simulink library "MOST_Lib"  (R2020b)
settings: Solver=VariableStepAuto  StartTime=0.0  StopTime=10.0  RelTol=1e-3
undefined symbols (not defined in the file): simu, wind, windTurbine, windturbine, X, Y, Z
libraries: nesl_utility x54, sm_lib x50, simulink x4, simulink_extras x1, pid_lib x1, WECSim_Lib_Body_Elements x1
(part 2 of 3)

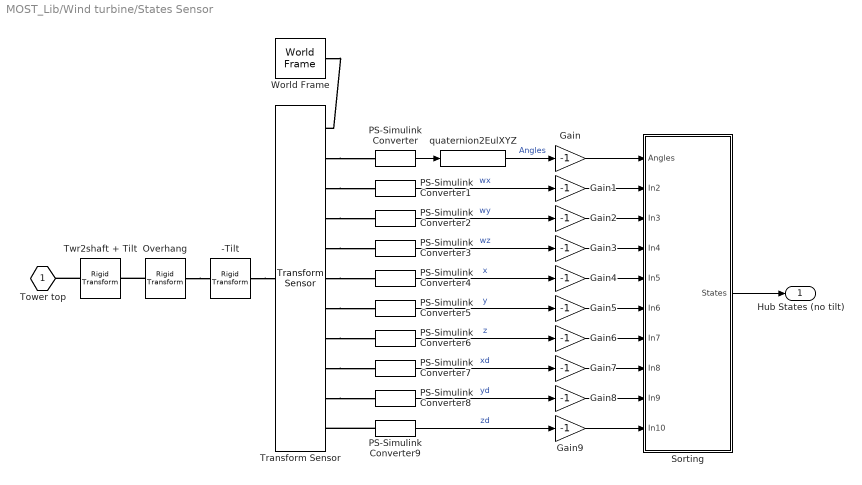
== system MOST_Lib/Wind turbine/States Sensor ==
  -Tilt : sm_lib/Frames and Transforms/Rigid Transform  RotationMethod=StandardAxis  FollAlignAxisA=+X  BaseAlignAxisA=+Y  FollAlignAxisB=+Y  BaseAlignAxisB=+Z  RotationStandardAxis=+Y  RotationAngle=-windTurbine.nacelle.tiltangle  RotationAngleUnits=deg  RotationArbitraryAxis=[0 0 1]  RotationSequenceAxes=FollowerAxes  RotationSequence=XYX  RotationSequenceAngles=[0 0 0]  RotationSequenceAnglesUnits=deg  RotationMatrix=[1 0 0; 0 1 0; 0 0 1]  Quaternion=[1 0 0 0]  TranslationMethod=None  TranslationCartesianOffset=[0 0 0]  TranslationCartesianOffsetUnits=m  TranslationStandardAxis=+Z  TranslationStandardOffset=0  TranslationStandardOffsetUnits=m  TranslationROffset=0  TranslationROffsetUnits=m  TranslationThetaOffset=0  TranslationThetaOffsetUnits=deg  TranslationZOffset=0  TranslationZOffsetUnits=m
  Gain{,1..9} (10 alike) : Gain  Gain=-1
  Overhang : sm_lib/Frames and Transforms/Rigid Transform  RotationMethod=None  FollAlignAxisA=+X  BaseAlignAxisA=+Y  FollAlignAxisB=+Y  BaseAlignAxisB=+Z  RotationStandardAxis=+Z  RotationAngle=0.0  RotationAngleUnits=deg  RotationArbitraryAxis=[0 0 1]  RotationSequenceAxes=FollowerAxes  RotationSequence=XYX  RotationSequenceAngles=[0 0 0]  RotationSequenceAnglesUnits=deg  RotationMatrix=[1 0 0; 0 1 0; 0 0 1]  Quaternion=[1 0 0 0]  TranslationMethod=StandardAxis  TranslationCartesianOffset=[0 0 0]  TranslationCartesianOffsetUnits=m  TranslationStandardAxis=+X  TranslationStandardOffset=windTurbine.hub.overhang  TranslationStandardOffsetUnits=m  TranslationROffset=0  TranslationROffsetUnits=m  TranslationThetaOffset=0  TranslationThetaOffsetUnits=deg  TranslationZOffset=0  TranslationZOffsetUnits=m
  PS-Simulink Converter{,1..9} (10 alike) : nesl_utility/PS-Simulink Converter  PhysicalDomain=network_engine_domain  SubClassName=ps_output  LeftPortType=input  RightPortType=output  PseudoPeriodic=off  Frequencies=[]  VectorFormat=inherit  Unit=inherit  AffineConversion=off
  Sorting : Subsystem
  Transform Sensor : sm_lib/Frames and Transforms/Transform Sensor  MeasurementFrame=World  RotationSequence=XYZ  SenseAngle=off  SenseAxis=off  SenseQ=on  SenseR=off  SenseRotationSequence=off  SenseOmegaX=on  SenseOmegaY=on  SenseOmegaZ=on  SenseOmega=off  SenseQDot=off  SenseRDot=off  SenseRotationSequenceDot=off  SenseAlphaX=off  SenseAlphaY=off  SenseAlphaZ=off  SenseAlpha=off  SenseQDDot=off  SenseRDDot=off  SenseX=on  SenseY=on  SenseZ=on  SenseXYZ=off  SenseRad=off  SenseAzim=off  SenseDist=off  SenseInc=off  SenseXDot=on  SenseYDot=on  SenseZDot=on  SenseXYZDot=off  SenseRadDot=off  SenseAzimDot=off  SenseDistDot=off  SenseIncDot=off  SenseXDDot=off  SenseYDDot=off  SenseZDDot=off  SenseXYZDDot=off  SenseRadDDot=off  SenseAzimDDot=off  SenseDistDDot=off  SenseIncDDot=off
  "Twr2shaft + Tilt " : sm_lib/Frames and Transforms/Rigid Transform  RotationMethod=StandardAxis  FollAlignAxisA=+X  BaseAlignAxisA=+Y  FollAlignAxisB=+Y  BaseAlignAxisB=+Z  RotationStandardAxis=+Y  RotationAngle=windTurbine.nacelle.tiltangle  RotationAngleUnits=deg  RotationArbitraryAxis=[0 0 1]  RotationSequenceAxes=FollowerAxes  RotationSequence=XYX  RotationSequenceAngles=[0 0 0]  RotationSequenceAnglesUnits=deg  RotationMatrix=[1 0 0; 0 1 0; 0 0 1]  Quaternion=[1 0 0 0]  TranslationMethod=StandardAxis  TranslationCartesianOffset=[0 0 0]  TranslationCartesianOffsetUnits=m  TranslationStandardAxis=+Z  TranslationStandardOffset=windTurbine.nacelle.Twr2Shft  TranslationStandardOffsetUnits=m  TranslationROffset=0  TranslationROffsetUnits=m  TranslationThetaOffset=0  TranslationThetaOffsetUnits=deg  TranslationZOffset=0  TranslationZOffsetUnits=m
  World Frame : sm_lib/Frames and Transforms/World Frame
  quaternion2EulXYZ : WECSim_Lib_Body_Elements/Rigid Body/Hydrodynamic Body/Structure/Motion Sensor/quaternion2EulXYZ  SystemSampleTime=-1  VariantActivationTime=update diagram  Latency=0  AutoFrameSizeCalculation=off
  Tower top : PMIOPort  Side=Left
  Hub States (no tilt) : Outport
  wires:
  PS-Simulink Converter/1 -> quaternion2EulXYZ/1
  quaternion2EulXYZ/1 -> Gain/1  "Angles"
  PS-Simulink Converter1/1 -> Gain1/1  "wx"
  PS-Simulink Converter2/1 -> Gain2/1  "wy"
  PS-Simulink Converter3/1 -> Gain3/1  "wz"
  PS-Simulink Converter4/1 -> Gain4/1  "x"
  PS-Simulink Converter5/1 -> Gain5/1  "y"
  PS-Simulink Converter6/1 -> Gain6/1  "z"
  PS-Simulink Converter7/1 -> Gain7/1  "xd"
  PS-Simulink Converter8/1 -> Gain8/1  "yd"
  PS-Simulink Converter9/1 -> Gain9/1  "zd"
  Sorting/1(States) -> Hub States (no tilt)/1
  Gain/1 -> Sorting/1(Angles)
  Gain1/1 -> Sorting/2(In2)
  Gain2/1 -> Sorting/3(In3)
  Gain3/1 -> Sorting/4(In4)
  Gain4/1 -> Sorting/5(In5)
  Gain5/1 -> Sorting/6(In6)
  Gain6/1 -> Sorting/7(In7)
  Gain7/1 -> Sorting/8(In8)
  Gain8/1 -> Sorting/9(In9)
  Gain9/1 -> Sorting/10(In10)
  connections:
  Transform Sensor/RConn7 -- PS-Simulink Converter5/LConn1
  World Frame/RConn1 -- Transform Sensor/RConn1
  "Twr2shaft + Tilt "/LConn1 -- Tower top/RConn1
  Transform Sensor/RConn2 -- PS-Simulink Converter/LConn1
  Transform Sensor/RConn3 -- PS-Simulink Converter1/LConn1
  Transform Sensor/RConn4 -- PS-Simulink Converter2/LConn1
  Transform Sensor/RConn5 -- PS-Simulink Converter3/LConn1
  Transform Sensor/RConn6 -- PS-Simulink Converter4/LConn1
  Transform Sensor/RConn9 -- PS-Simulink Converter7/LConn1
  Transform Sensor/RConn8 -- PS-Simulink Converter6/LConn1
  Transform Sensor/RConn10 -- PS-Simulink Converter8/LConn1
  PS-Simulink Converter9/LConn1 -- Transform Sensor/RConn11
  -Tilt/RConn1 -- Transform Sensor/LConn1
  Overhang/RConn1 -- -Tilt/LConn1
  Overhang/LConn1 -- "Twr2shaft + Tilt "/RConn1

== system MOST_Lib/Wind turbine/Tower ==
  Body Properties Tower : sm_lib/Body Elements/File Solid  ExtGeomFileName=geometry/NREL5MW_Tower.STL  UnitType=Custom  ExtGeomFileUnits=m  StepReaderType=HEX  ExportConvexHullGeometry=off  InertiaType=Custom  BasedOnType=Density  Density=1000  DensityUnits=kg/(m^3)  Mass=windTurbine.tower.mass  MassUnits=kg  CenterOfMass=[0 0 0]  CenterOfMassUnits=m  MomentsOfInertia=windTurbine.tower.inertia  MomentsOfInertiaUnits=kg*m^2  ProductsOfInertia=windTurbine.tower.inertiaProducts  ProductsOfInertiaUnits=kg*m^2  GraphicType=FromGeometry  MarkerShape=Sphere  MarkerSize=10  GraphicVisPropType=SimpleVisualProperties  GraphicDiffuseColor=[1 1 1]  GraphicOpacity=1  GraphicSpecularColor=[0.5 0.5 0.5 1.0]  GraphicAmbientColor=[0.15 0.15 0.15 1.0]  GraphicEmissiveColor=[0.0 0.0 0.0 1.0]  GraphicShininess=75  DoExposeReferenceFrame=on  SerializedFrames=<Frames/>
  Constant : Constant  Value=-windTurbine.tower.mass*simu.gravity
  External Force and Torque : sm_lib/Forces and Torques/External Force and Torque  EnableForceX=off  EnableForceY=off  EnableForceZ=on  EnableForce=off  ForceResolutionFrame=World  EnableTorqueX=off  EnableTorqueY=off  EnableTorqueZ=off  EnableTorque=off  TorqueResolutionFrame=AttachedFrame
  Relative COG Tower : sm_lib/Frames and Transforms/Rigid Transform  RotationMethod=None  FollAlignAxisA=+X  BaseAlignAxisA=+Y  FollAlignAxisB=+Y  BaseAlignAxisB=+Z  RotationStandardAxis=+Y  RotationAngle=0.05  RotationAngleUnits=rad  RotationArbitraryAxis=[0.57735026918962584 0.57735026918962584 0.57735026918962584]  RotationSequenceAxes=FollowerAxes  RotationSequence=XYX  RotationSequenceAngles=[0 0 0]  RotationSequenceAnglesUnits=deg  RotationMatrix=[1 0 0; 0 1 0; 0 0 1]  Quaternion=[1 0 0 0]  TranslationMethod=Cartesian  TranslationCartesianOffset=windTurbine.tower.cog_rel  TranslationCartesianOffsetUnits=m  TranslationStandardAxis=+Z  TranslationStandardOffset=0  TranslationStandardOffsetUnits=m  TranslationROffset=0  TranslationROffsetUnits=m  TranslationThetaOffset=0  TranslationThetaOffsetUnits=deg  TranslationZOffset=0  TranslationZOffsetUnits=m
  Simulink-PS Converter : nesl_utility/Simulink-PS Converter  PhysicalDomain=network_engine_domain  SubClassName=ps_input  LeftPortType=input  RightPortType=output  PseudoPeriodic=off  Frequencies=[]  NoiseDistribution=none  NoiseParameters=[]  Unit=1  AffineConversion=off  FilteringAndDerivatives=provide  SimscapeFilterOrder=1  InputFilterTimeConstant=0.001  UdotUserProvided=0
  Tower Base : PMIOPort  Side=Left
  wires:
  Constant/1 -> Simulink-PS Converter/1
  connections:
  Simulink-PS Converter/RConn1 -- External Force and Torque/LConn1
  Relative COG Tower/LConn1 -- Tower Base/RConn1
  Body Properties Tower/RConn1 -- Relative COG Tower/RConn1 -- External Force and Torque/RConn1

== system MOST_Lib/Wind turbine/TowerBaseLoad ==
  Mux : Mux  Inputs=2
  PS-Simulink Converter6 : nesl_utility/PS-Simulink Converter  PhysicalDomain=network_engine_domain  SubClassName=ps_output  LeftPortType=input  RightPortType=output  PseudoPeriodic=off  Frequencies=[]  VectorFormat=1-D array  Unit=inherit  AffineConversion=off
  PS-Simulink Converter7 : nesl_utility/PS-Simulink Converter  PhysicalDomain=network_engine_domain  SubClassName=ps_output  LeftPortType=input  RightPortType=output  PseudoPeriodic=off  Frequencies=[]  VectorFormat=1-D array  Unit=inherit  AffineConversion=off
  fc : PMIOPort  Side=Left
  tc : PMIOPort  Port=2  Side=Left
  tag scope: TowerBaseLoad1=global
  wires:
  PS-Simulink Converter7/1 -> Mux/1
  PS-Simulink Converter6/1 -> Mux/2
  Mux/1 -> [TowerBaseLoad1]
  connections:
  fc/RConn1 -- PS-Simulink Converter7/LConn1
  tc/RConn1 -- PS-Simulink Converter6/LConn1

== system MOST_Lib/Wind turbine/TowerTopLoad and deltaYaw ==
  Mux1 : Mux  Inputs=2
  PS-Simulink Converter1 : nesl_utility/PS-Simulink Converter  PhysicalDomain=network_engine_domain  SubClassName=ps_output  LeftPortType=input  RightPortType=output  PseudoPeriodic=off  Frequencies=[]  VectorFormat=1-D array  Unit=rad  AffineConversion=off
  PS-Simulink Converter8 : nesl_utility/PS-Simulink Converter  PhysicalDomain=network_engine_domain  SubClassName=ps_output  LeftPortType=input  RightPortType=output  PseudoPeriodic=off  Frequencies=[]  VectorFormat=1-D array  Unit=inherit  AffineConversion=off
  PS-Simulink Converter9 : nesl_utility/PS-Simulink Converter  PhysicalDomain=network_engine_domain  SubClassName=ps_output  LeftPortType=input  RightPortType=output  PseudoPeriodic=off  Frequencies=[]  VectorFormat=1-D array  Unit=inherit  AffineConversion=off
  q : PMIOPort  Side=Left
  ft : PMIOPort  Port=2  Side=Left
  tt : PMIOPort  Port=3  Side=Left
  tag scope: DeltaYaw1=global, TowerTopLoad1=global
  wires:
  PS-Simulink Converter9/1 -> Mux1/1
  PS-Simulink Converter8/1 -> Mux1/2
  Mux1/1 -> [TowerTopLoad1]
  PS-Simulink Converter1/1 -> [DeltaYaw1]
  connections:
  ft/RConn1 -- PS-Simulink Converter9/LConn1
  tt/RConn1 -- PS-Simulink Converter8/LConn1
  q/RConn1 -- PS-Simulink Converter1/LConn1

== system MOST_Lib/Wind turbine/Aerodynamics + Control/Aeroloads ==
  note: 1) Add Subsystem or Model blocks as valid variant choices.
      | 2) You cannot connect blocks at this level. At simulation, connectivity is automatically
      | determined, based on the active variant and port name matching.
  Aeroloads_in : Inport
  BEM : Subsystem  VariantControl=sv_t1_AeroLoads1
  Look-up Tables : Subsystem  VariantControl=sv_t1_AeroLoads0
  F_aero : Outport

== system MOST_Lib/Wind turbine/Aerodynamics + Control/Control ==
  note: 1) Add Subsystem or Model blocks as valid variant choices.
      | 2) You cannot connect blocks at this level. At simulation, connectivity is automatically
      | determined, based on the active variant and port name matching.
  Rotor speed : Inport
  Baseline : Subsystem  VariantControl=sv_t1_control0
  ROSCO : Subsystem  VariantControl=sv_t1_control1
  Gen torque : Outport
  Bladepitch : Outport  Port=2

== system MOST_Lib/Wind turbine/Aerodynamics + Control/Yaw Control ==
  Hub states (no tilt) : Inport
  Atan : Trigonometry  Operator=atan2  OutputSignalType=real
  Constant : Constant  Value=windTurbine.YawControlFlag
  Constant1 : Constant  Value=0
  Demux : Demux  Outputs=3
  Integrator : Integrator
  PID Controller : pid_lib/PID Controller  Controller=PID  Form=Parallel  TimeDomain=Continuous-time  UseExternalTs=off  SampleTime=-1  IntegratorMethod=Forward Euler  FilterMethod=Forward Euler  ControllerParametersSource=internal  P=windTurbine.YawControl.Kp  I=windTurbine.YawControl.Ki  D=windTurbine.YawControl.Kd  N=100  UseFilter=on  TunerSelectOption=Transfer Function Based (PID Tuner App)  InitialConditionSource=internal  InitialConditionForIntegrator=0  InitialConditionForFilter=0  DifferentiatorICPrevScaledInput=0  ExternalReset=none  TrackingMode=off  Kt=1  LimitOutput=on  SatLimitsSource=internal  UpperSaturationLimit=windTurbine.YawControl.maxYawRate  LowerSaturationLimit=-windTurbine.YawControl.maxYawRate  LinearizeAsGain=on  AntiWindupMode=clamping  Kb=1  POutMin=[]  POutMax=[]  IOutMin=[]  IOutMax=[]  DOutMin=[]  DOutMax=[]  NOutMin=[]  NOutMax=[]  SumOutMin=[]  SumOutMax=[]  SaturationOutMin=[]  SaturationOutMax=[]  PParamMin=[]  PParamMax=[]  IParamMin=[]  IParamMax=[]  DParamMin=[]  DParamMax=[]  NParamMin=[]  NParamMax=[]  KbParamMin=[]  KbParamMax=[]  KtParamMin=[]  KtParamMax=[]  KbOutMin=[]  KbOutMax=[]  KtOutMin=[]  KtOutMax=[]  IntegratorOutMin=[]  IntegratorOutMax=[]  FilterOutMin=[]  FilterOutMax=[]  SumI1OutMin=[]  SumI1OutMax=[]  SumI2OutMin=[]  SumI2OutMax=[]  SumI3OutMin=[]  SumI3OutMax=[]  SumI4OutMin=[]  SumI4OutMax=[]  SumDOutMin=[]  SumDOutMax=[]  DifferentiatorOutMin=[]  DifferentiatorOutMax=[]  FilterDiffOutCoefMin=[]  FilterDiffOutCoefMax=[]  ReciprocalOutMin=[]  ReciprocalOutMax=[]  SumDenOutMin=[]  SumDenOutMax=[]  SumNumOutMin=[]  SumNumOutMax=[]  DivideOutMin=[]  DivideOutMax=[]  UdiffTsProdOutMin=[]  UdiffTsProdOutMax=[]  NTsProdOutMin=[]  NTsProdOutMax=[]  UintegralTsProdOutMin=[]  UintegralTsProdOutMax=[]  UngainTsProdOutMin=[]  UngainTsProdOutMax=[]  IntegratorContinuousStateAttributes=''  IntegratorStateMustResolveToSignalObject=off  IntegratorRTWStateStorageClass=Auto  FilterContinuousStateAttributes=''  FilterStateMustResolveToSignalObject=off  FilterRTWStateStorageClass=Auto  ParallelPVariant=InternalParameters  IdealPVariant=Disabled  IVariant=InternalParameters  DVariant=InternalParameters  IntegratorVariant=Continuous  SatVariant=Enabled  AWVariant=ContClampingParallel  PCopyVariant=Disabled  TRVariant=Disabled  FdbkBlocksVariant=Forward  IdealPFdbkVariant=Disabled  SatFdbkVariant=Disabled  DerivativeFilterVariant=ContFilter  NVariant=InternalParameters  NCopyVariant=Disabled  FilterICVariant=InternalICsFilter  IntegratorICVariant=InternalICs  ExternalResetVariant=Disabled  TRSumVariant=Passthrough  SumFdbkVariant=Disabled  SumVariant=Sum_PID  TsampFilterVariant=InternalTs  TsampNgainVariant=Passthrough  TsampIntegralVariant=Disabled_SignalSpec  ExternalSaturationOutDataTypeStr=Inherit: Same as second input
  Selector : Selector  InputPortWidth=12  IndexOptions=Index vector (dialog)  Indices=[6]  OutputSizes=1
  Sum : Sum  Inputs=+|-
  Switch : Switch  Criteria=u2 > Threshold
  Terminator : Terminator
  Transfer Fcn : TransferFcn  Denominator=[windTurbine.YawControl.tau_system 1]
  DeltaYaw : Outport
  wires:
  Hub states (no tilt)/1 -> Selector/1
  Selector/1 -> Sum/2  "Hub Yaw (fb)"
  [WindSpeed1] -> Demux/1  "m/s"
  Demux/3 -> Terminator/1
  Demux/2 -> Atan/1
  Demux/1 -> Atan/2
  Atan/1 -> Sum/1  "wind xy angle (set)"
  Integrator/1 -> Switch/1
  Transfer Fcn/1 -> Integrator/1
  PID Controller/1 -> Transfer Fcn/1
  Sum/1 -> PID Controller/1
  Constant/1 -> Switch/2
  Constant1/1 -> Switch/3
  Switch/1 -> DeltaYaw/1

== system MOST_Lib/Wind turbine/Blade 1/Blade ==
  Body Properties Blade : sm_lib/Body Elements/File Solid  ExtGeomFileName=geometry/NREL5MW_Blade.STL  UnitType=Custom  ExtGeomFileUnits=m  StepReaderType=HEX  ExportConvexHullGeometry=off  InertiaType=Custom  BasedOnType=Density  Density=1000  DensityUnits=kg/(m^3)  Mass=windTurbine.blade.mass  MassUnits=kg  CenterOfMass=[0 0 0]  CenterOfMassUnits=m  MomentsOfInertia=windTurbine.blade.inertia  MomentsOfInertiaUnits=kg*m^2  ProductsOfInertia=windTurbine.blade.inertiaProducts  ProductsOfInertiaUnits=kg*m^2  GraphicType=FromGeometry  MarkerShape=Sphere  MarkerSize=10  GraphicVisPropType=SimpleVisualProperties  GraphicDiffuseColor=[1 1 1]  GraphicOpacity=1  GraphicSpecularColor=[0.5 0.5 0.5 1.0]  GraphicAmbientColor=[0.15 0.15 0.15 1.0]  GraphicEmissiveColor=[0.0 0.0 0.0 1.0]  GraphicShininess=75  DoExposeReferenceFrame=on  SerializedFrames=<Frames/>
  Constant : Constant  Value=-windTurbine.blade.mass*simu.gravity
  External Force and Torque : sm_lib/Forces and Torques/External Force and Torque  EnableForceX=off  EnableForceY=off  EnableForceZ=on  EnableForce=off  ForceResolutionFrame=World  EnableTorqueX=off  EnableTorqueY=off  EnableTorqueZ=off  EnableTorque=off  TorqueResolutionFrame=AttachedFrame
  Relative COG Blade : sm_lib/Frames and Transforms/Rigid Transform  RotationMethod=None  FollAlignAxisA=+X  BaseAlignAxisA=+Y  FollAlignAxisB=+Y  BaseAlignAxisB=+Z  RotationStandardAxis=+Y  RotationAngle=0.05  RotationAngleUnits=rad  RotationArbitraryAxis=[0.57735026918962584 0.57735026918962584 0.57735026918962584]  RotationSequenceAxes=FollowerAxes  RotationSequence=XYX  RotationSequenceAngles=[0 0 0]  RotationSequenceAnglesUnits=deg  RotationMatrix=[1 0 0; 0 1 0; 0 0 1]  Quaternion=[1 0 0 0]  TranslationMethod=Cartesian  TranslationCartesianOffset=windTurbine.blade.cog_rel  TranslationCartesianOffsetUnits=m  TranslationStandardAxis=+Z  TranslationStandardOffset=0  TranslationStandardOffsetUnits=m  TranslationROffset=0  TranslationROffsetUnits=m  TranslationThetaOffset=0  TranslationThetaOffsetUnits=deg  TranslationZOffset=0  TranslationZOffsetUnits=m
  Simulink-PS Converter : nesl_utility/Simulink-PS Converter  PhysicalDomain=network_engine_domain  SubClassName=ps_input  LeftPortType=input  RightPortType=output  PseudoPeriodic=off  Frequencies=[]  NoiseDistribution=none  NoiseParameters=[]  Unit=1  AffineConversion=off  FilteringAndDerivatives=provide  SimscapeFilterOrder=1  InputFilterTimeConstant=0.001  UdotUserProvided=0
  Blade Root : PMIOPort  Side=Left
  wires:
  Constant/1 -> Simulink-PS Converter/1
  connections:
  Relative COG Blade/RConn1 -- Body Properties Blade/RConn1 -- External Force and Torque/RConn1
  Relative COG Blade/LConn1 -- Blade Root/RConn1
  Simulink-PS Converter/RConn1 -- External Force and Torque/LConn1

== system MOST_Lib/Wind turbine/Blade 1/bladeRootLoad ==
  Mux : Mux  Inputs=2
  PS-Simulink Converter5 : nesl_utility/PS-Simulink Converter  PhysicalDomain=network_engine_domain  SubClassName=ps_output  LeftPortType=input  RightPortType=output  PseudoPeriodic=off  Frequencies=[]  VectorFormat=1-D array  Unit=inherit  AffineConversion=off
  PS-Simulink Converter6 : nesl_utility/PS-Simulink Converter  PhysicalDomain=network_engine_domain  SubClassName=ps_output  LeftPortType=input  RightPortType=output  PseudoPeriodic=off  Frequencies=[]  VectorFormat=1-D array  Unit=inherit  AffineConversion=off
  fc : PMIOPort  Side=Left
  tc : PMIOPort  Port=2  Side=Left
  tag scope: blade1RootLoad1=global
  wires:
  PS-Simulink Converter6/1 -> Mux/2
  Mux/1 -> [blade1RootLoad1]
  PS-Simulink Converter5/1 -> Mux/1
  connections:
  tc/RConn1 -- PS-Simulink Converter6/LConn1
  fc/RConn1 -- PS-Simulink Converter5/LConn1

== system MOST_Lib/Wind turbine/Blade 2/Blade ==
  Body Properties Blade : sm_lib/Body Elements/File Solid  ExtGeomFileName=geometry/NREL5MW_Blade.STL  UnitType=Custom  ExtGeomFileUnits=m  StepReaderType=HEX  ExportConvexHullGeometry=off  InertiaType=Custom  BasedOnType=Density  Density=1000  DensityUnits=kg/(m^3)  Mass=windTurbine.blade.mass  MassUnits=kg  CenterOfMass=[0 0 0]  CenterOfMassUnits=m  MomentsOfInertia=windTurbine.blade.inertia  MomentsOfInertiaUnits=kg*m^2  ProductsOfInertia=windTurbine.blade.inertiaProducts  ProductsOfInertiaUnits=kg*m^2  GraphicType=FromGeometry  MarkerShape=Sphere  MarkerSize=10  GraphicVisPropType=SimpleVisualProperties  GraphicDiffuseColor=[1 1 1]  GraphicOpacity=1  GraphicSpecularColor=[0.5 0.5 0.5 1.0]  GraphicAmbientColor=[0.15 0.15 0.15 1.0]  GraphicEmissiveColor=[0.0 0.0 0.0 1.0]  GraphicShininess=75  DoExposeReferenceFrame=on  SerializedFrames=<Frames/>
  Constant : Constant  Value=-windTurbine.blade.mass*simu.gravity
  External Force and Torque : sm_lib/Forces and Torques/External Force and Torque  EnableForceX=off  EnableForceY=off  EnableForceZ=on  EnableForce=off  ForceResolutionFrame=World  EnableTorqueX=off  EnableTorqueY=off  EnableTorqueZ=off  EnableTorque=off  TorqueResolutionFrame=AttachedFrame
  Relative COG Blade : sm_lib/Frames and Transforms/Rigid Transform  RotationMethod=None  FollAlignAxisA=+X  BaseAlignAxisA=+Y  FollAlignAxisB=+Y  BaseAlignAxisB=+Z  RotationStandardAxis=+Y  RotationAngle=0.05  RotationAngleUnits=rad  RotationArbitraryAxis=[0.57735026918962584 0.57735026918962584 0.57735026918962584]  RotationSequenceAxes=FollowerAxes  RotationSequence=XYX  RotationSequenceAngles=[0 0 0]  RotationSequenceAnglesUnits=deg  RotationMatrix=[1 0 0; 0 1 0; 0 0 1]  Quaternion=[1 0 0 0]  TranslationMethod=Cartesian  TranslationCartesianOffset=windTurbine.blade.cog_rel  TranslationCartesianOffsetUnits=m  TranslationStandardAxis=+Z  TranslationStandardOffset=0  TranslationStandardOffsetUnits=m  TranslationROffset=0  TranslationROffsetUnits=m  TranslationThetaOffset=0  TranslationThetaOffsetUnits=deg  TranslationZOffset=0  TranslationZOffsetUnits=m
  Simulink-PS Converter : nesl_utility/Simulink-PS Converter  PhysicalDomain=network_engine_domain  SubClassName=ps_input  LeftPortType=input  RightPortType=output  PseudoPeriodic=off  Frequencies=[]  NoiseDistribution=none  NoiseParameters=[]  Unit=1  AffineConversion=off  FilteringAndDerivatives=provide  SimscapeFilterOrder=1  InputFilterTimeConstant=0.001  UdotUserProvided=0
  Blade Root : PMIOPort  Side=Left
  wires:
  Constant/1 -> Simulink-PS Converter/1
  connections:
  Simulink-PS Converter/RConn1 -- External Force and Torque/LConn1
  Relative COG Blade/LConn1 -- Blade Root/RConn1
  External Force and Torque/RConn1 -- Body Properties Blade/RConn1 -- Relative COG Blade/RConn1

== system MOST_Lib/Wind turbine/Blade 2/bladeRootLoad ==
  Mux : Mux  Inputs=2
  PS-Simulink Converter5 : nesl_utility/PS-Simulink Converter  PhysicalDomain=network_engine_domain  SubClassName=ps_output  LeftPortType=input  RightPortType=output  PseudoPeriodic=off  Frequencies=[]  VectorFormat=1-D array  Unit=inherit  AffineConversion=off
  PS-Simulink Converter6 : nesl_utility/PS-Simulink Converter  PhysicalDomain=network_engine_domain  SubClassName=ps_output  LeftPortType=input  RightPortType=output  PseudoPeriodic=off  Frequencies=[]  VectorFormat=1-D array  Unit=inherit  AffineConversion=off
  fc : PMIOPort  Side=Left
  tc : PMIOPort  Port=2  Side=Left
  tag scope: blade2RootLoad1=global
  wires:
  PS-Simulink Converter5/1 -> Mux/1
  Mux/1 -> [blade2RootLoad1]
  PS-Simulink Converter6/1 -> Mux/2
  connections:
  fc/RConn1 -- PS-Simulink Converter5/LConn1
  tc/RConn1 -- PS-Simulink Converter6/LConn1

== system MOST_Lib/Wind turbine/Blade 3/Blade ==
  Body Properties Blade : sm_lib/Body Elements/File Solid  ExtGeomFileName=geometry/NREL5MW_Blade.STL  UnitType=Custom  ExtGeomFileUnits=m  StepReaderType=HEX  ExportConvexHullGeometry=off  InertiaType=Custom  BasedOnType=Density  Density=1000  DensityUnits=kg/(m^3)  Mass=windTurbine.blade.mass  MassUnits=kg  CenterOfMass=[0 0 0]  CenterOfMassUnits=m  MomentsOfInertia=windTurbine.blade.inertia  MomentsOfInertiaUnits=kg*m^2  ProductsOfInertia=windTurbine.blade.inertiaProducts  ProductsOfInertiaUnits=kg*m^2  GraphicType=FromGeometry  MarkerShape=Sphere  MarkerSize=10  GraphicVisPropType=SimpleVisualProperties  GraphicDiffuseColor=[1 1 1]  GraphicOpacity=1  GraphicSpecularColor=[0.5 0.5 0.5 1.0]  GraphicAmbientColor=[0.15 0.15 0.15 1.0]  GraphicEmissiveColor=[0.0 0.0 0.0 1.0]  GraphicShininess=75  DoExposeReferenceFrame=on  SerializedFrames=<Frames/>
  Constant : Constant  Value=-windTurbine.blade.mass*simu.gravity
  External Force and Torque : sm_lib/Forces and Torques/External Force and Torque  EnableForceX=off  EnableForceY=off  EnableForceZ=on  EnableForce=off  ForceResolutionFrame=World  EnableTorqueX=off  EnableTorqueY=off  EnableTorqueZ=off  EnableTorque=off  TorqueResolutionFrame=AttachedFrame
  Relative COG Blade : sm_lib/Frames and Transforms/Rigid Transform  RotationMethod=None  FollAlignAxisA=+X  BaseAlignAxisA=+Y  FollAlignAxisB=+Y  BaseAlignAxisB=+Z  RotationStandardAxis=+Y  RotationAngle=0.05  RotationAngleUnits=rad  RotationArbitraryAxis=[0.57735026918962584 0.57735026918962584 0.57735026918962584]  RotationSequenceAxes=FollowerAxes  RotationSequence=XYX  RotationSequenceAngles=[0 0 0]  RotationSequenceAnglesUnits=deg  RotationMatrix=[1 0 0; 0 1 0; 0 0 1]  Quaternion=[1 0 0 0]  TranslationMethod=Cartesian  TranslationCartesianOffset=windTurbine.blade.cog_rel  TranslationCartesianOffsetUnits=m  TranslationStandardAxis=+Z  TranslationStandardOffset=0  TranslationStandardOffsetUnits=m  TranslationROffset=0  TranslationROffsetUnits=m  TranslationThetaOffset=0  TranslationThetaOffsetUnits=deg  TranslationZOffset=0  TranslationZOffsetUnits=m
  Simulink-PS Converter : nesl_utility/Simulink-PS Converter  PhysicalDomain=network_engine_domain  SubClassName=ps_input  LeftPortType=input  RightPortType=output  PseudoPeriodic=off  Frequencies=[]  NoiseDistribution=none  NoiseParameters=[]  Unit=1  AffineConversion=off  FilteringAndDerivatives=provide  SimscapeFilterOrder=1  InputFilterTimeConstant=0.001  UdotUserProvided=0
  Blade Root : PMIOPort  Side=Left
  wires:
  Constant/1 -> Simulink-PS Converter/1
  connections:
  Simulink-PS Converter/RConn1 -- External Force and Torque/LConn1
  Relative COG Blade/LConn1 -- Blade Root/RConn1
  External Force and Torque/RConn1 -- Body Properties Blade/RConn1 -- Relative COG Blade/RConn1

== system MOST_Lib/Wind turbine/Blade 3/bladeRootLoad ==
  Mux : Mux  Inputs=2
  PS-Simulink Converter5 : nesl_utility/PS-Simulink Converter  PhysicalDomain=network_engine_domain  SubClassName=ps_output  LeftPortType=input  RightPortType=output  PseudoPeriodic=off  Frequencies=[]  VectorFormat=1-D array  Unit=inherit  AffineConversion=off
  PS-Simulink Converter6 : nesl_utility/PS-Simulink Converter  PhysicalDomain=network_engine_domain  SubClassName=ps_output  LeftPortType=input  RightPortType=output  PseudoPeriodic=off  Frequencies=[]  VectorFormat=1-D array  Unit=inherit  AffineConversion=off
  fc : PMIOPort  Side=Left
  tc : PMIOPort  Port=2  Side=Left
  tag scope: blade3RootLoad1=global
  wires:
  PS-Simulink Converter5/1 -> Mux/1
  Mux/1 -> [blade3RootLoad1]
  PS-Simulink Converter6/1 -> Mux/2
  connections:
  fc/RConn1 -- PS-Simulink Converter5/LConn1
  tc/RConn1 -- PS-Simulink Converter6/LConn1

== system MOST_Lib/Wind turbine/States Sensor/Sorting ==
  Angles : Inport
  In2 : Inport  Port=2
  In3 : Inport  Port=3
  In4 : Inport  Port=4
  In5 : Inport  Port=5
  In6 : Inport  Port=6
  In7 : Inport  Port=7
  In8 : Inport  Port=8
  In9 : Inport  Port=9
  In10 : Inport  Port=10
  Mux : Mux  Inputs=10
  States : Outport
  wires:
  In5/1 -> Mux/1  "x"
  In6/1 -> Mux/2  "y"
  Mux/1 -> States/1
  In3/1 -> Mux/9  "wy"
  In2/1 -> Mux/8  "wx"
  In7/1 -> Mux/3  "z"
  In8/1 -> Mux/5  "xd"
  Angles/1 -> Mux/4  "Ang"
  In9/1 -> Mux/6  "yd"
  In10/1 -> Mux/7  "zd"
  In4/1 -> Mux/10  "wz"

== system MOST_Lib/Wind turbine/Aerodynamics + Control/Aeroloads/BEM ==
  Aeroloads_in : Inport
  BEM : MATLAB Function  TreatAsAtomicUnit=on
  From Workspace3 : FromWorkspace  VariableName=wind.Input  OutputAfterFinalValue=Holding final value
  Hub wind speed : Subsystem
  Selector : Selector  InputPortWidth=15  IndexOptions=Index vector (dialog)  Indices=[1:14]  OutputSizes=1
  Selector1 : Selector  InputPortWidth=15  IndexOptions=Index vector (dialog)  Indices=[15]  OutputSizes=1
  F_aero : Outport
  wires:
  From Workspace3/1 -> Hub wind speed/1(wind_input), BEM/1(wind)
  BEM/1(F_aero_r_bl) -> F_aero/1
  Selector/1 -> BEM/2(q)
  Aeroloads_in/1 -> Selector1/1, Selector/1
  Selector1/1 -> BEM/3(bladepitch)

== system MOST_Lib/Wind turbine/Aerodynamics + Control/Aeroloads/Look-up Tables ==
  Aeroloads_in : Inport
  LUT : Subsystem
  Relative Wind : Subsystem
  Selector : Selector  InputPortWidth=15  IndexOptions=Index vector (dialog)  Indices=[15]  OutputSizes=1
  Selector1 : Selector  InputPortWidth=15  IndexOptions=Index vector (dialog)  Indices=[1:14]  OutputSizes=1
  Selector2 : Selector  InputPortWidth=15  IndexOptions=Index vector (dialog)  Indices=[14]  OutputSizes=1
  F_aero : Outport  PortDimensions=[6 3]
  wires:
  Aeroloads_in/1 -> Selector1/1, Selector2/1, Selector/1
  Selector/1 -> LUT/1(Bladepitch)  "Bladepitch"
  Selector2/1 -> LUT/3(Rotor speed)  "Rotor Speed"
  LUT/1(F_aero) -> F_aero/1
  Relative Wind/1(Relative Wind) -> LUT/2(Wind speed)
  Selector1/1 -> Relative Wind/1(q)  "q"

== system MOST_Lib/Wind turbine/Aerodynamics + Control/Control/Baseline ==
  Rotor speed : Inport
  " " : StateSpace  A=windTurbine.Baseline.omegaFilter.A  B=windTurbine.Baseline.omegaFilter.B  C=windTurbine.Baseline.omegaFilter.C  D=windTurbine.Baseline.omegaFilter.D  InitialCondition=[0,windTurbine.omega0/windTurbine.Baseline.omegaFilter.C(2)]
  Bladepitch control : Subsystem
  "Rate Limiter " : RateLimiter  RisingSlewLimit=windTurbine.Baseline.torqueMaxRate  FallingSlewLimit=-windTurbine.Baseline.torqueMaxRate  SampleTimeMode=inherited
  Torque control : Lookup_n-D  NumberOfTableDimensions=1  BreakpointsForDimension1=windTurbine.Baseline.omega_gen  Table=windTurbine.Baseline.Cgen  RndMeth=Simplest  InputSameDT=on
  Gen torque : Outport
  Bladepitch : Outport  Port=2
  wires:
  " "/1 -> Torque control/1, Bladepitch control/1(Rotor speed)
  Rotor speed/1 -> " "/1
  Torque control/1 -> "Rate Limiter "/1  "Nm"
  Bladepitch control/1(Bladepitch) -> Bladepitch/1  "rad"
  "Rate Limiter "/1 -> Gen torque/1  "Nm"

== system MOST_Lib/Wind turbine/Aerodynamics + Control/Control/ROSCO ==
  Rotor speed : Inport
  "ROSCO controller " : Subsystem
  Selector : Selector  InputPortWidth=3  IndexOptions=Index vector (dialog)  Indices=[1]  OutputSizes=1
  Gen torque : Outport
  Bladepitch : Outport  Port=2
  wires:
  Rotor speed/1 -> "ROSCO controller "/1(Generator speed)  "rad/s"
  [NacXdot1] -> "ROSCO controller "/3(NacXdot)  "m/s"
  "ROSCO controller "/2(Bladepitch) -> Bladepitch/1  "rad"
  [WindSpeed1] -> Selector/1  "m/s"
  "ROSCO controller "/1(Gen torque) -> Gen torque/1  "Nm"
  Selector/1 -> "ROSCO controller "/2(Wind speed)  "m/s"

== system MOST_Lib/Wind turbine/Aerodynamics + Control/Aeroloads/BEM/Hub wind speed ==
  wind_input : Inport
  Constant1 : Constant  Value=windTurbine.hub.height
  Constant2 : Constant  Value=windTurbine.offset_plane
  Demux : Demux  Outputs=2
  Mux : Mux  Inputs=3
  Selector : Selector  NumberOfDimensions=4  InputPortWidth=3  IndexOptions=Select all,Select all,Select all,Index vector (dialog)  Indices=[1 3],1,1,1  OutputSizes=1,1,1,1
  Selector1 : Selector  NumberOfDimensions=4  InputPortWidth=3  IndexOptions=Select all,Select all,Select all,Index vector (dialog)  Indices=[1 3],1,1,2  OutputSizes=1,1,1,1
  Selector2 : Selector  NumberOfDimensions=4  InputPortWidth=3  IndexOptions=Select all,Select all,Select all,Index vector (dialog)  Indices=[1 3],1,1,3  OutputSizes=1,1,1,1
  Wind : Lookup_n-D  NumberOfTableDimensions=3  BreakpointsForDimension1=wind.Xdiscr  BreakpointsForDimension2=wind.Ydiscr  BreakpointsForDimension3=wind.Zdiscr  BeginIndexSearchUsingPreviousIndexResult=on  TableSource=Input port  Table=permute(squeeze(wind.Input.signals.values(find(abs(wind.Xdiscr-0)==min(abs(wind.Xdiscr-0)),1),:,:,1,:)),[3 1 2])  InternalRulePriority=Speed  RndMeth=Simplest  InputSameDT=on
      settings: InputPortMap=u0,u1,u2,p221
  Wind1 : Lookup_n-D  NumberOfTableDimensions=3  BreakpointsForDimension1=wind.Xdiscr  BreakpointsForDimension2=wind.Ydiscr  BreakpointsForDimension3=wind.Zdiscr  BeginIndexSearchUsingPreviousIndexResult=on  TableSource=Input port  Table=permute(squeeze(wind.Input.signals.values(find(abs(wind.Xdiscr-0)==min(abs(wind.Xdiscr-0)),1),:,:,1,:)),[3 1 2])  InternalRulePriority=Speed  RndMeth=Simplest  InputSameDT=on
      settings: InputPortMap=u0,u1,u2,p221
  Wind2 : Lookup_n-D  NumberOfTableDimensions=3  BreakpointsForDimension1=wind.Xdiscr  BreakpointsForDimension2=wind.Ydiscr  BreakpointsForDimension3=wind.Zdiscr  BeginIndexSearchUsingPreviousIndexResult=on  TableSource=Input port  Table=permute(squeeze(wind.Input.signals.values(find(abs(wind.Xdiscr-0)==min(abs(wind.Xdiscr-0)),1),:,:,1,:)),[3 1 2])  InternalRulePriority=Speed  RndMeth=Simplest  InputSameDT=on
      settings: InputPortMap=u0,u1,u2,p221
  tag scope: WindSpeed1=global
  wires:
  Wind/1 -> Mux/1
  Mux/1 -> [WindSpeed1]
  Wind1/1 -> Mux/2
  Wind2/1 -> Mux/3
  Constant2/1 -> Demux/1
  Demux/1 -> Wind/1, Wind2/1, Wind1/1
  Constant1/1 -> Wind/3, Wind1/3, Wind2/3
  wind_input/1 -> Selector2/1, Selector1/1, Selector/1
  Selector/1 -> Wind/4
  Selector1/1 -> Wind1/4
  Selector2/1 -> Wind2/4
  Demux/2 -> Wind/2, Wind1/2, Wind2/2

== system MOST_Lib/Wind turbine/Aerodynamics + Control/Aeroloads/Look-up Tables/LUT ==
  Bladepitch : Inport
  Wind speed : Inport  Port=2
  Rotor speed : Inport  Port=3
  For Iterator Subsystem : Subsystem  TreatAsAtomicUnit=on
  F_aero : Outport  PortDimensions=[6 3]
  wires:
  Wind speed/1 -> For Iterator Subsystem/1(Wind speed)
  Rotor speed/1 -> For Iterator Subsystem/2(Rotor speed)
  Bladepitch/1 -> For Iterator Subsystem/3(Bladepitch)
  For Iterator Subsystem/1(F_aero) -> F_aero/1

== system MOST_Lib/Wind turbine/Aerodynamics + Control/Aeroloads/Look-up Tables/Relative Wind ==
  q : Inport
  Calc Relative Wind : MATLAB Function  TreatAsAtomicUnit=on
  Constant : Constant  Value=windTurbine.nacelle.tiltangle*pi/180
  Constant1 : Constant  Value=windTurbine.hub.precone*pi/180
  Constant3 : Constant  Value=windTurbine.blade.bladeDiscr
  Constant4 : Constant  Value=wind.Xdiscr
  Constant5 : Constant  Value=windTurbine.blade.BlCrvAC
  Constant6 : Constant  Value=windTurbine.blade.BlSwpAC
  Constant7 : Constant  Value=windTurbine.blade.BlCrvAng
  Constant8 : Constant  Value=wind.Ydiscr
  Constant9 : Constant  Value=wind.Zdiscr
  From Workspace3 : FromWorkspace  VariableName=wind.Input  OutputAfterFinalValue=Holding final value
  Hub wind speed : Subsystem
  Relative Wind : Outport
  wires:
  Calc Relative Wind/1(v_wind_rel_bl_x) -> Relative Wind/1
  q/1 -> Calc Relative Wind/2(q)
  Constant/1 -> Calc Relative Wind/3(tilt)
  Constant1/1 -> Calc Relative Wind/4(precone)
  Constant3/1 -> Calc Relative Wind/5(bladeDiscr)
  Constant5/1 -> Calc Relative Wind/6(BlCrvAC)
  Constant7/1 -> Calc Relative Wind/8(BlCrvAng)
  Constant6/1 -> Calc Relative Wind/7(BlSwpAC)
  From Workspace3/1 -> Hub wind speed/1(wind_input), Calc Relative Wind/1(wind)
  Constant4/1 -> Calc Relative Wind/9(Wind_Xdiscr)
  Constant8/1 -> Calc Relative Wind/10(Wind_Ydiscr)
  Constant9/1 -> Calc Relative Wind/11(Wind_Zdiscr)

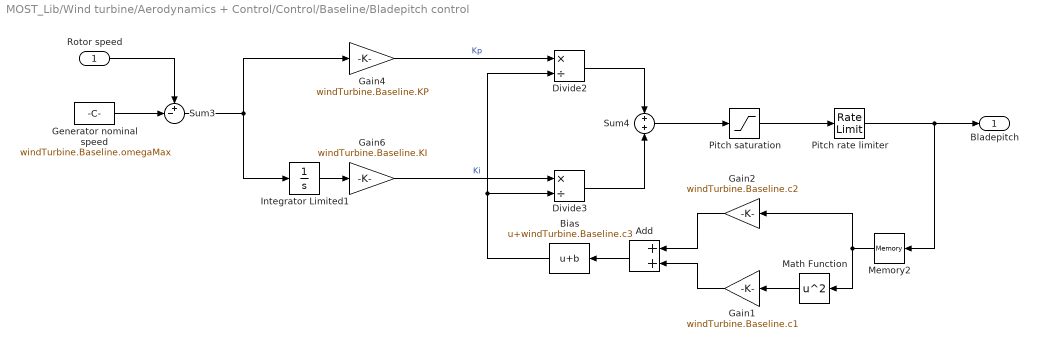
== system MOST_Lib/Wind turbine/Aerodynamics + Control/Control/Baseline/Bladepitch control ==
  Rotor speed : Inport
  Add : Sum
  Bias : Bias  Bias=windTurbine.Baseline.c3
  Divide2 : Product  Inputs=*/
  Divide3 : Product  Inputs=*/
  Gain1 : Gain  Gain=windTurbine.Baseline.c1
  Gain2 : Gain  Gain=windTurbine.Baseline.c2
  Gain4 : Gain  Gain=windTurbine.Baseline.KP
  Gain6 : Gain  Gain=windTurbine.Baseline.KI
  Generator nominal speed : Constant  Value=windTurbine.Baseline.omegaMax
  Integrator Limited1 : Integrator  LimitOutput=on  LowerSaturationLimit=0
  Math Function : Math  Operator=square  SaturateOnIntegerOverflow=on
  Memory2 : Memory  InitialCondition=windTurbine.bladepitch0
  Pitch rate limiter : RateLimiter  RisingSlewLimit=windTurbine.Baseline.thetaMaxRate  FallingSlewLimit=-windTurbine.Baseline.thetaMaxRate  SampleTimeMode=inherited  InitialCondition=windTurbine.bladepitch0
  Pitch saturation : Saturate  UpperLimit=pi/2  LowerLimit=0
  Sum3 : Sum  Inputs=+-|
  Sum4 : Sum
  Bladepitch : Outport  VectorParamsAs1DForOutWhenUnconnected=off
  wires:
  Integrator Limited1/1 -> Gain6/1
  Bias/1 -> Divide3/2, Divide2/2
  Add/1 -> Bias/1
  Sum4/1 -> Pitch saturation/1
  Generator nominal speed/1 -> Sum3/2
  Pitch rate limiter/1 -> Bladepitch/1, Memory2/1
  Pitch saturation/1 -> Pitch rate limiter/1
  Gain6/1 -> Divide3/1  "Ki"
  Sum3/1 -> Gain4/1, Integrator Limited1/1
  Gain4/1 -> Divide2/1  "Kp"
  Divide3/1 -> Sum4/2
  Divide2/1 -> Sum4/1
  Rotor speed/1 -> Sum3/1
  Gain1/1 -> Add/2
  Gain2/1 -> Add/1
  Math Function/1 -> Gain1/1
  Memory2/1 -> Math Function/1, Gain2/1

== system MOST_Lib/Wind turbine/Aerodynamics + Control/Control/ROSCO/ROSCO controller  ==
  Generator speed : Inport
  Wind speed : Inport  Port=2
  NacXdot : Inport  Port=3
  " " : StateSpace  A=windTurbine.ROSCO.omegaFilter.A  B=windTurbine.ROSCO.omegaFilter.B  C=windTurbine.ROSCO.omegaFilter.C  D=windTurbine.ROSCO.omegaFilter.D  InitialCondition=[0,(0*pi/30)/windTurbine.ROSCO.omegaFilter.C(2)]
  "  " : StateSpace  A=windTurbine.ROSCO.windFilter.A  B=windTurbine.ROSCO.windFilter.B  C=windTurbine.ROSCO.windFilter.C  D=windTurbine.ROSCO.windFilter.D  InitialCondition=[0,0/windTurbine.ROSCO.windFilter.C(2)]
  Bladepitch control : Subsystem
  Setpoint smoother : Subsystem
  Torque control : Subsystem
  Transfer Fcn : TransferFcn  Denominator=[windTurbine.ROSCO.pitchFilter.A windTurbine.ROSCO.pitchFilter.B 1]
  Gen torque : Outport
  Bladepitch : Outport  Port=2
  wires:
  Wind speed/1 -> "  "/1
  Bladepitch control/1(Bladepitch) -> Bladepitch/1, Setpoint smoother/2(Bladepitch)
  NacXdot/1 -> Transfer Fcn/1
  Torque control/1(Gen torque) -> Gen torque/1, Setpoint smoother/1(Gen torque)
  Transfer Fcn/1 -> Bladepitch control/4(NacXdot)
  Generator speed/1 -> " "/1
  Setpoint smoother/1(Del_Omega_g) -> Bladepitch control/1(Del_Omega_g), Torque control/3(Del_omega_g)
  " "/1 -> Bladepitch control/3(Gen speed), Torque control/1(Gen speed)
  "  "/1 -> Torque control/2(Wind speed), Bladepitch control/2(Wind speed)

== system MOST_Lib/Wind turbine/Aerodynamics + Control/Aeroloads/Look-up Tables/LUT/For Iterator Subsystem ==
  Wind speed : Inport
  Rotor speed : Inport  Port=2
  Bladepitch : Inport  Port=3
  " " : Subsystem
  For Iterator : ForIterator  IterationLimit=6
  F_aero : Outport
  wires:
  Wind speed/1 -> " "/1(Wind speed)
  Rotor speed/1 -> " "/2(Rotor speed)
  Bladepitch/1 -> " "/3(Bladepitch)
  " "/1(F_aero) -> F_aero/1
  For Iterator/1 -> " "/4(Index)

== system MOST_Lib/Wind turbine/Aerodynamics + Control/Aeroloads/Look-up Tables/Relative Wind/Hub wind speed ==
  wind_input : Inport
  Constant1 : Constant  Value=windTurbine.hub.height
  Constant2 : Constant  Value=windTurbine.offset_plane
  Demux : Demux  Outputs=2
  Mux : Mux  Inputs=3
  Selector : Selector  NumberOfDimensions=4  InputPortWidth=3  IndexOptions=Select all,Select all,Select all,Index vector (dialog)  Indices=[1 3],1,1,1  OutputSizes=1,1,1,1
  Selector1 : Selector  NumberOfDimensions=4  InputPortWidth=3  IndexOptions=Select all,Select all,Select all,Index vector (dialog)  Indices=[1 3],1,1,2  OutputSizes=1,1,1,1
  Selector2 : Selector  NumberOfDimensions=4  InputPortWidth=3  IndexOptions=Select all,Select all,Select all,Index vector (dialog)  Indices=[1 3],1,1,3  OutputSizes=1,1,1,1
  Wind : Lookup_n-D  NumberOfTableDimensions=3  BreakpointsForDimension1=wind.Xdiscr  BreakpointsForDimension2=wind.Ydiscr  BreakpointsForDimension3=wind.Zdiscr  BeginIndexSearchUsingPreviousIndexResult=on  TableSource=Input port  Table=permute(squeeze(wind.Input.signals.values(find(abs(wind.Xdiscr-0)==min(abs(wind.Xdiscr-0)),1),:,:,1,:)),[3 1 2])  InternalRulePriority=Speed  RndMeth=Simplest  InputSameDT=on
      settings: InputPortMap=u0,u1,u2,p221
  Wind1 : Lookup_n-D  NumberOfTableDimensions=3  BreakpointsForDimension1=wind.Xdiscr  BreakpointsForDimension2=wind.Ydiscr  BreakpointsForDimension3=wind.Zdiscr  BeginIndexSearchUsingPreviousIndexResult=on  TableSource=Input port  Table=permute(squeeze(wind.Input.signals.values(find(abs(wind.Xdiscr-0)==min(abs(wind.Xdiscr-0)),1),:,:,1,:)),[3 1 2])  InternalRulePriority=Speed  RndMeth=Simplest  InputSameDT=on
      settings: InputPortMap=u0,u1,u2,p221
  Wind2 : Lookup_n-D  NumberOfTableDimensions=3  BreakpointsForDimension1=wind.Xdiscr  BreakpointsForDimension2=wind.Ydiscr  BreakpointsForDimension3=wind.Zdiscr  BeginIndexSearchUsingPreviousIndexResult=on  TableSource=Input port  Table=permute(squeeze(wind.Input.signals.values(find(abs(wind.Xdiscr-0)==min(abs(wind.Xdiscr-0)),1),:,:,1,:)),[3 1 2])  InternalRulePriority=Speed  RndMeth=Simplest  InputSameDT=on
      settings: InputPortMap=u0,u1,u2,p221
  tag scope: WindSpeed1=global
  wires:
  Wind/1 -> Mux/1
  Mux/1 -> [WindSpeed1]
  Wind1/1 -> Mux/2
  Wind2/1 -> Mux/3
  Constant2/1 -> Demux/1
  Demux/1 -> Wind2/1, Wind1/1, Wind/1
  Constant1/1 -> Wind2/3, Wind1/3, Wind/3
  wind_input/1 -> Selector2/1, Selector1/1, Selector/1
  Selector/1 -> Wind/4
  Selector1/1 -> Wind1/4
  Selector2/1 -> Wind2/4
  Demux/2 -> Wind2/2, Wind1/2, Wind/2

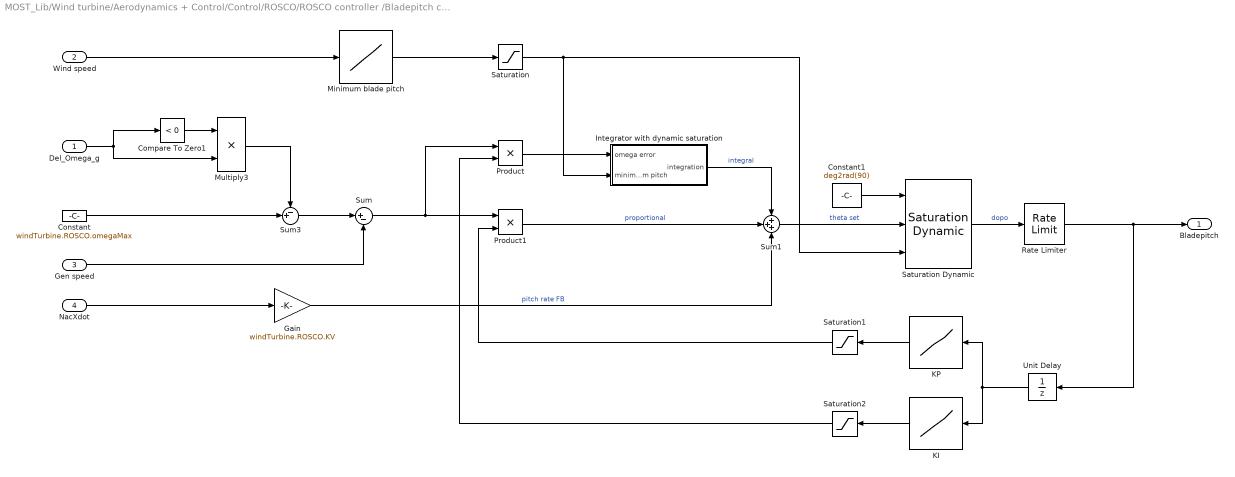
== system MOST_Lib/Wind turbine/Aerodynamics + Control/Control/ROSCO/ROSCO controller /Bladepitch control ==
  Del_Omega_g : Inport
  Wind speed : Inport  Port=2
  Gen speed : Inport  Port=3
  NacXdot : Inport  Port=4
  Compare To Zero1 : simulink/Logic and Bit Operations/Compare To Zero  relop=<  OutDataTypeStr=boolean
  Constant : Constant  Value=windTurbine.ROSCO.omegaMax
  Constant1 : Constant  Value=deg2rad(90)
  Gain : Gain  Gain=windTurbine.ROSCO.KV
  Integrator with dynamic saturation : Subsystem
  KI : Lookup_n-D  NumberOfTableDimensions=1  BreakpointsForDimension1=windTurbine.ROSCO.theta  Table=windTurbine.ROSCO.KI_theta  InternalRulePriority=Speed  RndMeth=Simplest  InputSameDT=on
  KP : Lookup_n-D  NumberOfTableDimensions=1  BreakpointsForDimension1=windTurbine.ROSCO.theta  Table=windTurbine.ROSCO.KP_theta  InternalRulePriority=Speed  RndMeth=Simplest  InputSameDT=on
  "Minimum blade pitch " : Lookup_n-D  NumberOfTableDimensions=1  BreakpointsForDimension1=windTurbine.ROSCO.WS  Table=windTurbine.ROSCO.MINBLADEPITCH  InternalRulePriority=Speed  RndMeth=Simplest  InputSameDT=on
  Multiply3 : Product
  Product : Product
  Product1 : Product
  "Rate Limiter " : RateLimiter  RisingSlewLimit=windTurbine.ROSCO.thetaMaxRate  FallingSlewLimit=-windTurbine.ROSCO.thetaMaxRate  SampleTimeMode=inherited  InitialCondition=windTurbine.bladepitch0
  Saturation : Saturate  UpperLimit=deg2rad(90)  LowerLimit=0
  "Saturation Dynamic " : simulink/Discontinuities/Saturation Dynamic  OutMin=[]  OutMax=[]  OutDataTypeStr=Inherit: Same as second input  OutDataType=fixdt(1, 16)  OutScaling=2^-10  DoSatur=off
  Saturation1 : Saturate  UpperLimit=windTurbine.ROSCO.KP_theta(end)  LowerLimit=windTurbine.ROSCO.KP_theta(1)
  Saturation2 : Saturate  UpperLimit=windTurbine.ROSCO.KI_theta(end)  LowerLimit=windTurbine.ROSCO.KI_theta(1)
  Sum : Sum  Inputs=|+-
  Sum1 : Sum  Inputs=+++
  Sum3 : Sum  Inputs=-+|
  Unit Delay : UnitDelay  InitialCondition=windTurbine.bladepitch0  SampleTime=-1  HasFrameUpgradeWarning=on
  Bladepitch : Outport
  wires:
  Saturation/1 -> "Saturation Dynamic "/3, Integrator with dynamic saturation/2(minimum pitch)
  "Rate Limiter "/1 -> Unit Delay/1, Bladepitch/1
  NacXdot/1 -> Gain/1
  "Saturation Dynamic "/1 -> "Rate Limiter "/1  "dopo"
  Sum3/1 -> Sum/1
  Constant/1 -> Sum3/2
  Del_Omega_g/1 -> Compare To Zero1/1, Multiply3/2
  Compare To Zero1/1 -> Multiply3/1
  Multiply3/1 -> Sum3/1
  KI/1 -> Saturation2/1
  KP/1 -> Saturation1/1
  Unit Delay/1 -> KI/1, KP/1
  Sum1/1 -> "Saturation Dynamic "/2  "theta set"
  Integrator with dynamic saturation/1(integration) -> Sum1/1  "integral"
  Product1/1 -> Sum1/2  "proportional"
  Sum/1 -> Product1/1, Product/1
  Product/1 -> Integrator with dynamic saturation/1(omega error)
  Constant1/1 -> "Saturation Dynamic "/1
  "Minimum blade pitch "/1 -> Saturation/1
  Wind speed/1 -> "Minimum blade pitch "/1
  Gen speed/1 -> Sum/2
  Saturation1/1 -> Product1/2
  Saturation2/1 -> Product/2
  Gain/1 -> Sum1/3  "pitch rate FB"

== system MOST_Lib/Wind turbine/Aerodynamics + Control/Control/ROSCO/ROSCO controller /Setpoint smoother ==
  Gen torque : Inport
  Bladepitch : Inport  Port=2
  Bias : Bias  Bias=-windTurbine.ROSCO.torqueMax
  Gain : Gain  Gain=windTurbine.ROSCO.SPS_kb/deg2rad(30)
  Gain1 : Gain  Gain=-windTurbine.ROSCO.SPS_kt/windTurbine.ROSCO.torqueMax
  Gain2 : Gain  Gain=windTurbine.ROSCO.omegaMax
  Sum2 : Sum  Inputs=+|-
  Transfer Fcn : TransferFcn  Denominator=[windTurbine.ROSCO.SPSFilter.A 1]
  Del_Omega_g : Outport  VectorParamsAs1DForOutWhenUnconnected=off
  wires:
  Gen torque/1 -> Bias/1
  Bladepitch/1 -> Gain/1
  Gain2/1 -> Del_Omega_g/1
  Bias/1 -> Gain1/1
  Sum2/1 -> Transfer Fcn/1
  Transfer Fcn/1 -> Gain2/1
  Gain/1 -> Sum2/1
  Gain1/1 -> Sum2/2

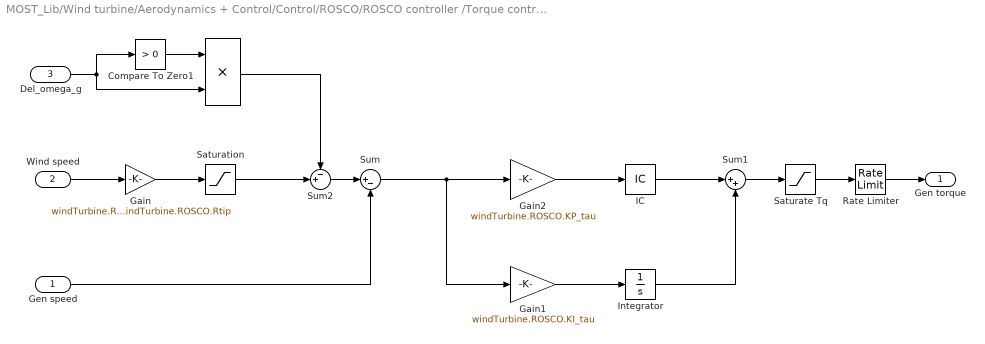
== system MOST_Lib/Wind turbine/Aerodynamics + Control/Control/ROSCO/ROSCO controller /Torque control ==
  Gen speed : Inport
  Wind speed : Inport  Port=2
  Del_omega_g : Inport  Port=3
  "  " : Product
  Compare To Zero1 : simulink/Logic and Bit Operations/Compare To Zero  relop=>  OutDataTypeStr=boolean
  Gain : Gain  Gain=windTurbine.ROSCO.TSR_opt/windTurbine.ROSCO.Rtip
  Gain1 : Gain  Gain=windTurbine.ROSCO.KI_tau
  Gain2 : Gain  Gain=windTurbine.ROSCO.KP_tau
  IC : InitialCondition  Value=0
  Integrator : Integrator  InitialCondition=windTurbine.GenTorque0  LimitOutput=on  UpperSaturationLimit=windTurbine.ROSCO.torqueMax  LowerSaturationLimit=0
  "Rate Limiter " : RateLimiter  RisingSlewLimit=windTurbine.ROSCO.torqueMaxRate  FallingSlewLimit=-windTurbine.ROSCO.torqueMaxRate  SampleTimeMode=inherited
  Saturate Tq : Saturate  UpperLimit=windTurbine.ROSCO.torqueMax  LowerLimit=0
  Saturation : Saturate  UpperLimit=windTurbine.ROSCO.omegaMax  LowerLimit=windTurbine.ROSCO.omegaMin
  Sum : Sum  Inputs=|+-
  Sum1 : Sum  Inputs=|++
  Sum2 : Sum  Inputs=-+|
  Gen torque : Outport
  wires:
  Integrator/1 -> Sum1/2
  Gain1/1 -> Integrator/1
  Gain2/1 -> IC/1
  Saturate Tq/1 -> "Rate Limiter "/1
  Sum2/1 -> Sum/1
  Del_omega_g/1 -> Compare To Zero1/1, "  "/2
  Compare To Zero1/1 -> "  "/1
  "  "/1 -> Sum2/1
  Sum/1 -> Gain2/1, Gain1/1
  Saturation/1 -> Sum2/2
  Gain/1 -> Saturation/1
  Sum1/1 -> Saturate Tq/1
  Gen speed/1 -> Sum/2
  Wind speed/1 -> Gain/1
  "Rate Limiter "/1 -> Gen torque/1
  IC/1 -> Sum1/1
